simulink model "myAdderROS"  (R2017b)
settings: Solver=FixedStepAuto  StartTime=0.0  StopTime=Inf  RelTol=1e-3
libraries: robotlib x4
settings Model: Creator=tkikawad  LastModifiedBy=tkikawad
settings OptimizationCC: PassReuseOutputArgsAs=Individual arguments  MaxStackSize=64
settings DebuggingCC: ParameterTunabilityLossMsg=error
settings HardwareCC: ProdBitPerLong=64  ProdHWDeviceType=Intel->x86-64 (Linux 64)
settings SFSimCC: MATLABDynamicMemAlloc=off
settings RTWCC: SystemTargetFile=ert.tlc  HardwareBoard=Robot Operating System (ROS)  GenCodeOnly=on  TemplateMakefile=ert_default_tmf  GenerateReport=on  Toolchain=Catkin  IncludeHyperlinkInReport=on  LaunchReport=on  TargetLang=C++  GenerateTraceInfo=on  GenerateTraceReport=on  GenerateTraceReportSl=on  GenerateTraceReportSf=on  GenerateTraceReportEml=on
settings CodeAppCC: ForceParamTrailComments=on  IgnoreCustomStorageClasses=off  OperatorAnnotations=on  SimulinkDataObjDesc=on  SFDataObjDesc=on  InsertBlockDesc=on

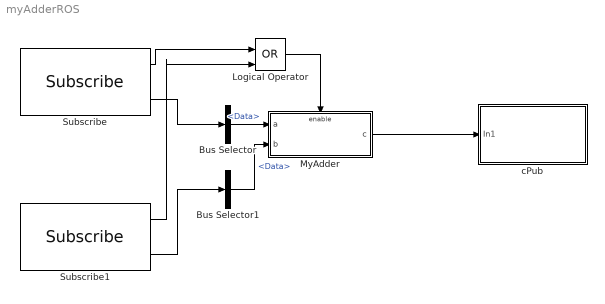
== system myAdderROS ==
  Bus Selector : BusSelector  OutputSignals=Data
  Bus Selector1 : BusSelector  OutputSignals=Data
  Logical Operator : Logic  Operator=OR  IconShape=distinctive  AllPortsSameDT=off  OutDataTypeStr=boolean
  MyAdder : Subsystem
  Subscribe : robotlib/Subscribe  SourceLibraryInfo=This block requires Robotics System Toolbox  topicSource=Specify your own  topic=/a  messageType=std_msgs/Float64  sampleTime=-1  messageQueueLength=1
      settings: SourceProductBaseCode=RO
  Subscribe1 : robotlib/Subscribe  SourceLibraryInfo=This block requires Robotics System Toolbox  topicSource=Specify your own  topic=/b  messageType=std_msgs/Float64  sampleTime=-1  messageQueueLength=1
      settings: SourceProductBaseCode=RO
  cPub : Subsystem
  wires:
  Subscribe1/2 -> Bus Selector1/1
  Subscribe1/1 -> Logical Operator/2
  Logical Operator/1 -> MyAdder/Enable
  Subscribe/1 -> Logical Operator/1
  Subscribe/2 -> Bus Selector/1
  Bus Selector/1 -> MyAdder/1(a)  "<Data>"
  Bus Selector1/1 -> MyAdder/2(b)  "<Data>"
  MyAdder/1(c) -> cPub/1(In1)

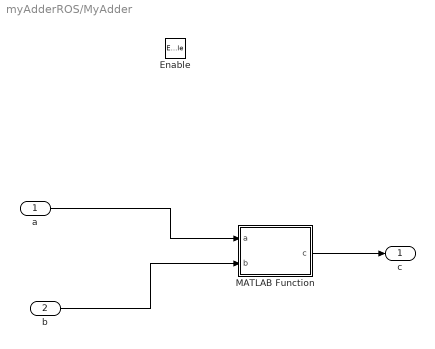
== system myAdderROS/MyAdder ==
  a : Inport
  b : Inport  Port=2
  Enable : EnablePort
  MATLAB Function : MATLAB Function  TreatAsAtomicUnit=on
  c : Outport
  wires:
  b/1 -> MATLAB Function/2(b)
  a/1 -> MATLAB Function/1(a)
  MATLAB Function/1(c) -> c/1

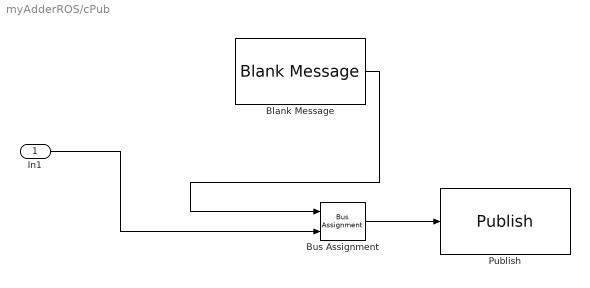
== system myAdderROS/cPub ==
  In1 : Inport
  Blank Message : robotlib/Blank Message  SourceLibraryInfo=This block requires Robotics System Toolbox  messageType=std_msgs/Float64  SampleTime=-1
      settings: SourceProductBaseCode=RO
  Bus Assignment : BusAssignment  AssignedSignals=Data
  Publish : robotlib/Publish  SourceLibraryInfo=This block requires Robotics System Toolbox  topicSource=Specify your own  topic=/c  messageType=std_msgs/Float64  messageQueueLength=1
      settings: SourceProductBaseCode=RO
  wires:
  In1/1 -> Bus Assignment/2
  Blank Message/1 -> Bus Assignment/1
  Bus Assignment/1 -> Publish/1

== matlab function myAdderROS/MyAdder/MATLAB Function ==
  data: a input; c output; b input
function c = fcn(a, b)
%#codegen
coder.inline('never');
c = 0;
c = myAdder(a,b);
